simulink model "Circuito_SM_I"  (R2025b)
settings: Solver=ode1  StartTime=0.0  StopTime=.1  FixedStep=1/100000  RelTol=1e-3  EnableMultiTasking=on
values from neighbouring files (symbols this model uses):
  N = 125000    [ExtraccionSimulacion.m]    (also in Fix4simErr.m; test4err.m)
undefined symbols (not defined in the file or in its folder): u2av
libraries: spsMosfetLib x4, spsPWMGeneratorDCDCLib x4, spsSeriesRLCBranchLib x3, spsIdealSwitchLib x2, spsControlledVoltageSourceLib x1, spsCurrentMeasurementLib x1, spsDCMachineLib x1, spsDCVoltageSourceLib x1, spsVoltageMeasurementLib x1, spspowerguiLib x1
settings Model: SimulationMode=rapid-accelerator  Creator=pepe  LastModifiedBy=Jorge
settings SolverCC: AlgebraicLoopSolver=TrustRegion  AutoInsertRateTranBlk=on
settings DataIOCC: LimitDataPoints=on  SaveFormat=Array  SignalLoggingSaveFormat=ModelDataLogs
settings OptimizationCC: ExpressionDepthLimit=2147483647.0  LifeSpan=inf
settings DebuggingCC: UnderspecifiedInitializationDetection=Classic  MergeDetectMultiDrivingBlocksExec=none  SolverPrmCheckMsg=warning  FcnCallInpInsideContextMsg=warning  UnconnectedInputMsg=warning  UnconnectedOutputMsg=warning  UnconnectedLineMsg=warning  StateNameClashWarn=warning  SFUnexpectedBacktrackingDiag=warning  SFNoUnconditionalDefaultTransitionDiag=warning  SFExecutionAtInitializationDiag=none  ArithmeticOperatorsInVariantConditions=warning
settings HardwareCC: ProdBitPerPointer=32.0  ProdBitPerSizeT=32.0  ProdBitPerPtrDiffT=32.0  ProdLargestAtomicFloat=None  ProdIntDivRoundTo=Undefined  ProdEndianess=Unspecified  ProdWordSize=32.0  ProdHWDeviceType=32-bit Generic
settings ModelReferenceCC: EnableRefExpFcnMdlSchedulingChecks=on  PropagateSignalLabelsOutOfModel=off
settings SFSimCC: SimUseLocalCustomCode=off  CustomCodeUndefinedFunction=UseInterfaceOnly
settings RTWCC: RTWUseLocalCustomCode=off  GPUComputeCapability=3.5
settings CodeAppCC: StateflowObjectComments=on
settings GRTTargetCC: TargetLangStandard=C89/C90 (ANSI)
settings ConfigComp: CovMetricSettings=dw  CovSaveCumulativeToWorkspaceVar=on  CovSaveSingleToWorkspaceVar=on  CovExternalEMLEnable=off
settings SimscapeCC: SimscapeNormalizeSystem=off

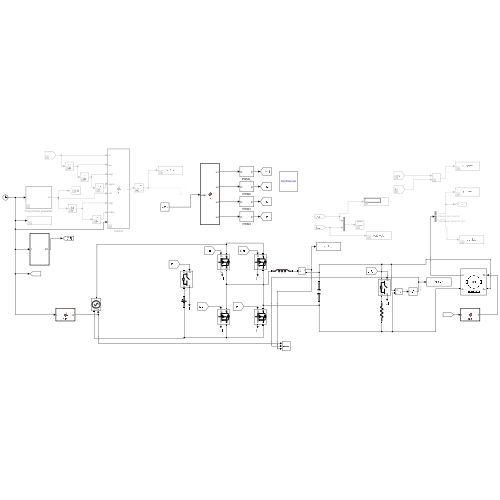
[thumbnail: Simulink's stored preview of the top-level diagram]
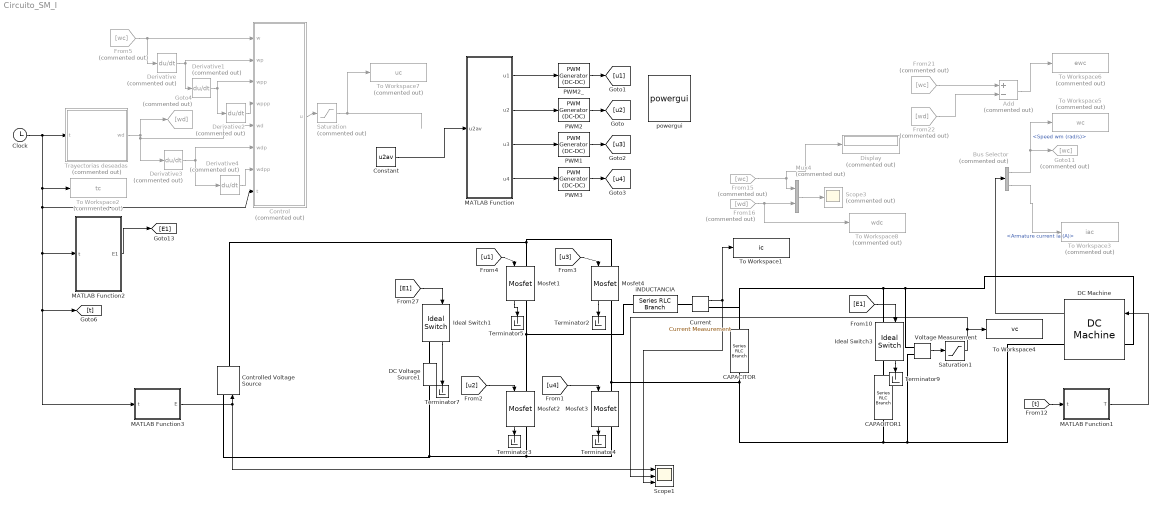
== system Circuito_SM_I ==
  Add : Sum  Commented=on  Inputs=+-
  Bus Selector : BusSelector  Commented=on  OutputSignals=Speed wm (rad/s),Armature current ia (A)
  CAPACITOR : spsSeriesRLCBranchLib/Series RLC Branch  LConnTagsString=__new0  RConnTagsString=__new0  BranchType=C  Resistance=1  Inductance=1e-3  SetiL0=off  InitialCurrent=0  Capacitance=114.4e-6  Setx0=off  InitialVoltage=45  Measurements=None
  CAPACITOR1 : spsSeriesRLCBranchLib/Series RLC Branch  LConnTagsString=__new0  RConnTagsString=__new0  BranchType=R  Resistance=64  Inductance=1e-3  SetiL0=off  InitialCurrent=0  Capacitance=114.4e-6  Setx0=off  InitialVoltage=45  Measurements=None
  Clock : Clock
  Constant : Constant  Value=u2av
  Control : MATLAB Function  Commented=on  TreatAsAtomicUnit=on
  Controlled Voltage Source : spsControlledVoltageSourceLib/Controlled Voltage Source  Initialize=on  Source_Type=DC  Amplitude=0  Phase=0  Frequency=0  Measurements=Voltage
  "Current " : spsCurrentMeasurementLib/Current Measurement  PhasorSimulation=off  OutputType=Complex  PSBequivalent=0
  DC Machine : spsDCMachineLib/DC Machine  PresetModel=No  MechanicalLoad=Torque TL  FieldType=Permanent magnet  ShowDetailedParameters=on  MeasurementBus=off  RLa="[ 0.965  0.00222]"  RLf="[ 240  120]"  Laf=1.8  MachineConstant=Torque constant (N.m/A)  Ke=10.94185305  Kt=1.74145  J=118.2e-3  Bm=129.6e-3  Tf=0  w0=0  Ifinit=0  TsPowergui=0  TsBlock=-1
  DC Voltage Source1 : spsDCVoltageSourceLib/DC Voltage Source  Amplitude=30  Measurements=None
  Derivative{,1..4} (5 alike) : Derivative  Commented=on
  Display : Display  Commented=on
  From15 : From  Commented=on  GotoTag=wc
  From16 : From  Commented=on  GotoTag=wd
  From21 : From  Commented=on  GotoTag=wc
  From22 : From  Commented=on  GotoTag=wd
  From5 : From  Commented=on  GotoTag=wc
  Goto11 : Goto  Commented=on  GotoTag=wc
  Goto4 : Goto  Commented=on  GotoTag=wd
  Ideal Switch1 : spsIdealSwitchLib/Ideal Switch  Ron=0.001  Lon=0  IC=0  Rs=1e5  Cs=inf  Measurements=on
  Ideal Switch3 : spsIdealSwitchLib/Ideal Switch  Ron=0.001  Lon=0  IC=0  Rs=1e5  Cs=inf  Measurements=on
  MATLAB Function : MATLAB Function  TreatAsAtomicUnit=on
  MATLAB Function1 : MATLAB Function  TreatAsAtomicUnit=on
  MATLAB Function2 : MATLAB Function  TreatAsAtomicUnit=on
  MATLAB Function3 : MATLAB Function  TreatAsAtomicUnit=on
  Mosfet{1..4} (4 alike) : spsMosfetLib/Mosfet  Ron=0  Lon=0  Rd=0.001  Vfd=0  IC=0  Rs=1e5  Cs=inf  Measurements=on
  Mux4 : Mux  Commented=on  Inputs=2
  PWM1 : spsPWMGeneratorDCDCLib/PWM Generator (DC-DC)  Fsw=50000  Ts=0
  PWM2 : spsPWMGeneratorDCDCLib/PWM Generator (DC-DC)  Fsw=50000  Ts=0
  PWM2_ : spsPWMGeneratorDCDCLib/PWM Generator (DC-DC)  Fsw=50000  Ts=0
  PWM3 : spsPWMGeneratorDCDCLib/PWM Generator (DC-DC)  Fsw=50000  Ts=0
  Saturation : Saturate  Commented=on  UpperLimit=1  LowerLimit=-1
  Saturation1 : Saturate  UpperLimit=30  LowerLimit=-30
  Scope1 : Scope  NumInputPorts=3
      settings: ActiveDisplayYMinimum=-6.3300692045441256  ActiveDisplayYMaximum=43.837890533392965
  Scope3 : Scope  Commented=on
      settings: ActiveDisplayYMinimum=-1.25  ActiveDisplayYMaximum=11.25  DataLoggingVariableName=ScopeData3
  Terminator{2..5,7,9} (6 alike) : Terminator
  To Workspace1 : ToWorkspace  VariableName=ic  SaveFormat=Timeseries  SampleTime=-1
      settings: Save2DSignal=2-D array (concatenate along first dimension)
  To Workspace2 : ToWorkspace  Commented=on  VariableName=tc  SampleTime=-1
  To Workspace3 : ToWorkspace  Commented=on  VariableName=iac  SampleTime=-1
  To Workspace4 : ToWorkspace  VariableName=vc  SaveFormat=Timeseries  SampleTime=-1
  To Workspace5 : ToWorkspace  Commented=on  VariableName=wc  SampleTime=-1
  To Workspace6 : ToWorkspace  Commented=on  VariableName=ewc  SampleTime=-1
  To Workspace7 : ToWorkspace  Commented=on  VariableName=uc  SampleTime=-1
  To Workspace8 : ToWorkspace  Commented=on  VariableName=wdc  SampleTime=-1
  Trayectorias deseadas : MATLAB Function  Commented=on  TreatAsAtomicUnit=on
  Voltage Measurement : spsVoltageMeasurementLib/Voltage Measurement  PhasorSimulation=off  OutputType=Complex  PSBequivalent=0
  iNDUCTANCIA : spsSeriesRLCBranchLib/Series RLC Branch  LConnTagsString=__new0  RConnTagsString=__new0  BranchType=L  Resistance=1  Inductance=15e-3  SetiL0=off  InitialCurrent=0  Capacitance=1e-6  Setx0=off  InitialVoltage=0  Measurements=None
  powergui : spspowerguiLib/powergui  Priority=1  SimulationMode=Continuous  SampleTime=50e-6  frequency=60  Iterations=50  frequencyindice=0  Pbase=100e6  ErrMax=1e-4  UnitsV=kV  UnitsW=MW  buscounter=0  FunctionMessages=off  echomessages=off  EnableUseOfTLC=off  CurrentSourceSwitches=off  DisableSnubberDevices=off  DisableRonSwitches=off  DisableVfSwitches=off  DisplayEquations=off  AutomaticDiscreteSolvers=off  SolverType=Tustin  Interpol=off  ExternalGateDelay=off  methode=off  Ts=0  x0status=blocks  SPID=on  SwTol=0  HookPort=off  NonlinearTolerance=1e-4  nMaxIteration=100  ContinueOnMaxIteration=off  RestoreLinks=warning  ResistiveCurrentMeasurement=off  Frange=[0:2:500]  Ylog=off  Xlog=on  ShowGrid=off  save=off  variable=ZData  structure=0  ZoomFFT=off  StartTime=0.0  cycles=1  DisplayStyle=1  fundamental=60  FreqAxis=off  MaxFrequency=1000  frequencyindicesteady=1  RmsSteady=1  display=off
  wires:
  [u4] -> Mosfet3/1
  Mosfet3/1 -> Terminator4/1
  Mosfet2/1 -> Terminator3/1
  [u2] -> Mosfet2/1
  Mosfet1/1 -> Terminator5/1
  Mosfet4/1 -> Terminator2/1
  [u3] -> Mosfet4/1
  [u1] -> Mosfet1/1
  Voltage Measurement/1 -> Saturation1/1
  DC Machine/1 -> Bus Selector/1
  MATLAB Function1/1(T) -> DC Machine/1
  MATLAB Function/1(u1) -> PWM2_/1
  MATLAB Function/2(u2) -> PWM2/1
  PWM2/1 -> [u2]
  PWM2_/1 -> [u1]
  PWM1/1 -> [u3]
  MATLAB Function/3(u3) -> PWM1/1
  PWM3/1 -> [u4]
  MATLAB Function/4(u4) -> PWM3/1
  Mux4/1 -> Scope3/1
  From16/1 -> To Workspace8/1, Mux4/2
  From15/1 -> Display/1, Mux4/1
  Bus Selector/1 -> To Workspace5/1, Goto11/1  "<Speed wm (rad/s)>"
  Bus Selector/2 -> To Workspace3/1  "<Armature current ia (A)>"
  Derivative/1 -> Derivative1/1, Control/2(wp)
  From5/1 -> Control/1(w), Derivative/1
  Derivative1/1 -> Derivative2/1, Control/3(wpp)
  Derivative4/1 -> Control/7(wdpp)
  Derivative2/1 -> Control/4(wppp)
  Control/1(u) -> Saturation/1
  Saturation/1 -> To Workspace7/1
  Derivative3/1 -> Derivative4/1, Control/6(wdp)
  Trayectorias deseadas/1(wd) -> Derivative3/1, Control/5(wd), Goto4/1
  Ideal Switch1/1 -> Terminator7/1
  [E1] -> Ideal Switch1/1
  MATLAB Function2/1(E1) -> [E1]
  Clock/1 -> MATLAB Function3/1(t), [t], MATLAB Function2/1(t), Control/8(t), To Workspace2/1, Trayectorias deseadas/1(t)
  [E1] -> Ideal Switch3/1
  [t] -> MATLAB Function1/1(t)
  From22/1 -> Add/2
  Add/1 -> To Workspace6/1
  From21/1 -> Add/1
  Ideal Switch3/1 -> Terminator9/1
  MATLAB Function3/1(E) -> Scope1/1, Controlled Voltage Source/1
  "Current "/1 -> Scope1/3, To Workspace1/1
  Saturation1/1 -> Scope1/2, To Workspace4/1
  Constant/1 -> MATLAB Function/1(u2av)
  connections:
  CAPACITOR/LConn1 -- "Current "/RConn1 -- Ideal Switch3/LConn1 -- Voltage Measurement/LConn1 -- DC Machine/LConn1
  iNDUCTANCIA/RConn1 -- "Current "/LConn1
  DC Voltage Source1/LConn1 -- Controlled Voltage Source/LConn1 -- Mosfet2/RConn1 -- Mosfet3/RConn1
  Mosfet3/LConn1 -- Mosfet4/RConn1 -- CAPACITOR1/RConn1 -- Voltage Measurement/LConn2 -- DC Machine/RConn1 -- CAPACITOR/RConn1
  Mosfet4/LConn1 -- Controlled Voltage Source/RConn1 -- Mosfet1/LConn1
  Mosfet2/LConn1 -- Mosfet1/RConn1 -- iNDUCTANCIA/LConn1
  Ideal Switch1/RConn1 -- DC Voltage Source1/RConn1
  Ideal Switch3/RConn1 -- CAPACITOR1/LConn1

== matlab function Circuito_SM_I/Control ==
  data: w input; wp input; u output; wpp input; wppp input; wd input; wdp input; wdpp input; t input
function u = fcn(w,wp,wpp,wppp,wd,wdp,wdpp,t)

%Parámetros
%E = 30;
E=3.3*(11.008+0.5504*sin(5*t)+0.5848*sin(10*t));
R = 64;
L = 15e-3;
C = 114.4e-6;
n = 14.5; 
Ra = 0.965;
La = 2.22e-3;
ke = 120.1e-3;
km = 120.1e-3;
J = 118.2e-3;
b = 129.6e-3;

%Ganancias
%A=2000;
%Lm=1000;
%k=2000000;

A=2000;
Lm=1000;
k=500000;

e=w-wd;

ep=wp-wdp;

epp=wpp-wdpp;

i=(J*La*C/(n*km))*wppp+((b*R*La*C+J*R*Ra*C+J*La)/(R*n*km))*wpp+((b*La+J*Ra+J*R+b*R*Ra*C+R*n*n*ke*km*C)/(n*km*R))*wp+((b*Ra+n*n*ke*km+b*R)/(n*km*R))*w;

v=((J*La)/(n*km))*wpp+((b*La+J*Ra)/(n*km))*wp+((b*Ra/(n*km))+n*ke)*w;

S=ep+Lm*e+A*L*i;

u=((-k*sign(S)-epp-Lm*ep)/(A*E))+(v/E);

== matlab function Circuito_SM_I/MATLAB Function ==
  data: u1 output; u2av input; u2 output; u3 output; u4 output
function [u1,u2,u3,u4] = fcn(u2av)
if u2av >= 0
    u1 = u2av;
    u2 = u2av*(-1);
    u3 = 0;
    u4 = 1;
else
   
    u1 = 0;
    u2 = 1;
    u3 = u2av*(-1);
    u4 = u2av;
end

== matlab function Circuito_SM_I/Trayectorias deseadas ==
  data: t input; wd output
function wd   = fcn(t)
%% Parámetro de la trayectoria senoidal
%% Tiempos para las trayectorias 
%     ti = 4; %4
%     tf = 6; %6 
%     t_div = (t-ti)/(tf-ti);
% % Valores deseados para las trayectorias
% %Velocidad
%     wi=10;
%     wf=-10;
% %% Polinomios de Bezier 
%  phi=0;
% if t <= ti
%     phi = 0;
% else
%     if t>ti && t<tf
%         phi = t_div^5*(252-1050*t_div+1800*t_div^2-1575*t_div^3+700*(t_div)^4-126*t_div^5);
%     else
%         if t>=tf
%             phi = 1;
%         end
%     end
% end
% wd = wi+phi*(wf-wi);
%wd=10;
 wd=10*sin(2*pi*t/2.5);

== matlab function Circuito_SM_I/MATLAB Function1 ==
  data: t input; T output
function T = fcn(t)
% 
% if t >= 2.5 && t < 5
%     T = -0.5;
% elseif t >= 7.5 && t < 10
%     T=0.5;
% else
%     T = 0;
% end

if t >= 2.5 && t < 5
    T = 0;
elseif t >= 7.5 && t < 10
    T=0;
else
    T = 0;
end

== matlab function Circuito_SM_I/MATLAB Function3 ==
  data: t input; E output
function E = fcn(t)

E=3.3*(11.008+0.5504*sin(5*t)+0.5848*sin(10*t));

== matlab function Circuito_SM_I/MATLAB Function2 ==
  data: E1 output; t input
function E1 = fcn(t)
% if t >= 2.5 && t < 5
%     E2 = 1;
%     E1 = 0;
%     E3 = 0;
% elseif t >= 7.5 && t < 10
%     E2 = 0;
%     E1 = 0;
%     E3 = 1;
% else
%     E2 = 0;
%     E1 = 1;
%     E3 = 0;
% end

if t >= 2.5 && t < 5
    E2 = 0;
    E1 = 1;
    E3 = 0;
elseif t >= 7.5 && t < 10
    E2 = 0;
    E1 = 1;
    E3 = 0;
else
    E2 = 0;
    E1 = 1;
    E3 = 0;
end
end
